simulink library "CalculateDistance_ul"  (R2018b)
settings: Solver=VariableStepAuto  StartTime=0.0  StopTime=10.0  RelTol=1e-3
settings Model: Creator=mcobb  LastModifiedBy=mae-ncsucore
settings DebuggingCC: LibraryContextMissingDiagnostic=none
settings SFSimCC: SimUseLocalCustomCode=off
settings RTWCC: RTWUseLocalCustomCode=off

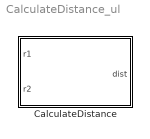
== system CalculateDistance_ul ==
  CalculateDistance : Subsystem

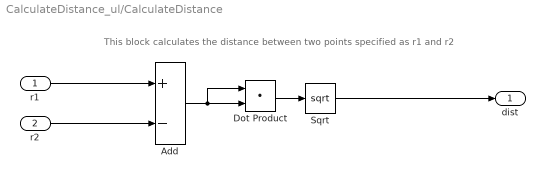
== system CalculateDistance_ul/CalculateDistance ==
  note: This block calculates the distance between two points specified as r1 and r2
  r1 : Inport
  r2 : Inport  Port=2
  Add : Sum  Inputs=+-
  Dot Product : DotProduct  InputSameDT=on  OutDataTypeStr=Inherit: Inherit via internal rule
  Sqrt : Sqrt  SaturateOnIntegerOverflow=on
  dist : Outport
  wires:
  Dot Product/1 -> Sqrt/1
  Add/1 -> Dot Product/2, Dot Product/1
  r2/1 -> Add/2
  r1/1 -> Add/1
  Sqrt/1 -> dist/1
